simulink model "torque_controller"  (R2014b)
settings: Solver=FixedStepDiscrete  StartTime=0.0  StopTime=inf  FixedStep=sample_time  RelTol=1e-3
StartFcn:
  | tg.sampletime = correctedSampleTime;
libraries: slrtlib x1
settings Model: SimulationMode=external  BufferReuse=off  Creator=wmartin  LastModifiedBy=drl
settings SolverCC: EnableConcurrentExecution=on
settings DataIOCC: LimitDataPoints=off  MaxDataPoints=1e7  SaveFormat=StructureWithTime  SignalLogging=off  DSMLogging=off
settings OptimizationCC: BlockReduction=off  OptimizeBlockIOStorage=off  BufferReuse=off  GlobalBufferReuse=off  ExpressionFolding=off  ExpressionDepthLimit=2147483647  LocalBlockOutputs=off  SimCompilerOptimization=On
settings DebuggingCC: UnderspecifiedInitializationDetection=Classic  MergeDetectMultiDrivingBlocksExec=none  StateNameClashWarn=warning
settings HardwareCC: ProdIntDivRoundTo=Zero  ProdEndianess=LittleEndian  ProdLongLongMode=on  ProdHWDeviceType=Generic->32-bit x86 compatible
settings ModelReferenceCC: UpdateModelReferenceTargets=IfOutOfDate  ModelReferenceNumInstancesAllowed=Single  ModelReferenceMinAlgLoopOccurrences=on
settings RTWCC: SystemTargetFile=slrt.tlc  TemplateMakefile=slrt_default_tmf  Description=Simulink Real-Time  RTWVerbose=off  ProcessScript=slrt_make_rtw_hook  RTWCompilerOptimization=On
settings CodeAppCC: MaxIdLength=256
settings SimulinkRealTimeCC: GeneratePreprocessorConditionals=Disable all  EnableShiftOperators=on  RL32LogBufSizeModifier=1e8

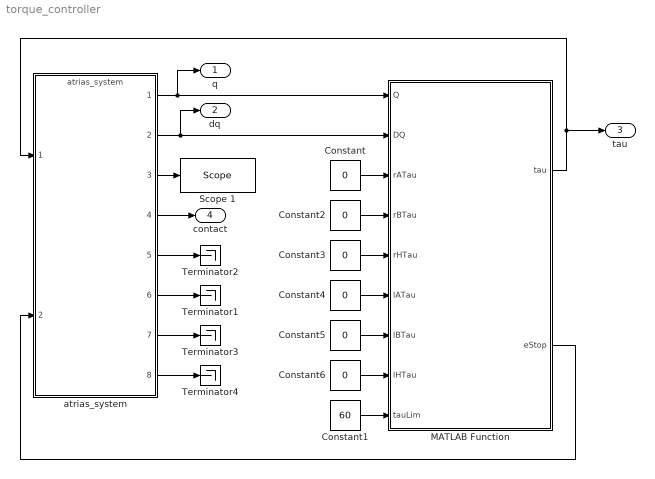
== system torque_controller ==
  Constant{,2..6} (6 alike) : Constant  Value=0
  Constant1 : Constant  Value=60
  MATLAB Function : MATLAB Function  TreatAsAtomicUnit=on
  Scope 1 : slrtlib/Displays and Logging/Scope   scopeno=1  scopetype=Target  autostart=on  viewmode=Graphical sliding  formatstr='%15.6f'  grid=on  ylimits=[0,0]  nosamples=5000  noprepostsamples=0  interleave=1  triggermode=FreeRun  triggersignal=1  trigsignalfromport=off  triggerlevel=0.0  triggerslope=Either  triggerscope=1  triggersample=0  filename=data.dat  mode=Lazy  writesize=512  autorestart=off  dynamicfilemode=off  maxwritefilesize=512*1024^2
  Terminator{1..4} (4 alike) : Terminator
  atrias_system : ModelReference  ModelNameDialog=atrias_system  SimulationMode=Normal  ModelReferenceVersion=1.2412  CopyOfModelName=atrias_system  DefaultDataLogging=on
  q : Outport
  dq : Outport  Port=2
  tau : Outport  Port=3
  contact : Outport  Port=4
  wires:
  atrias_system/2 -> dq/1, MATLAB Function/2(DQ)
  MATLAB Function/1(tau) -> tau/1, atrias_system/1
  MATLAB Function/2(eStop) -> atrias_system/2
  Constant/1 -> MATLAB Function/3(rATau)
  atrias_system/1 -> q/1, MATLAB Function/1(Q)
  Constant1/1 -> MATLAB Function/9(tauLim)
  Constant3/1 -> MATLAB Function/5(rHTau)
  Constant2/1 -> MATLAB Function/4(rBTau)
  Constant4/1 -> MATLAB Function/6(lATau)
  Constant5/1 -> MATLAB Function/7(lBTau)
  Constant6/1 -> MATLAB Function/8(lHTau)
  atrias_system/4 -> contact/1
  atrias_system/6 -> Terminator1/1
  atrias_system/7 -> Terminator3/1
  atrias_system/5 -> Terminator2/1
  atrias_system/8 -> Terminator4/1
  atrias_system/3 -> Scope 1/1

== matlab function torque_controller/MATLAB Function ==
  data: Q input; tau output; DQ input; rATau input; rBTau input; rHTau input; lATau input; lBTau input; lHTau input; eStop output; tauLim input
function [tau, eStop] = torqueController(Q, DQ, rATau, rBTau, rHTau, lATau, lBTau, lHTau, tauLim)
%TRACKINGCONTROLLER Trajectory tracking contoller.
%
% Description:
%
% Notes:
% 	- State indexes (rBl rBm rAl rAm lBl lBm lAl lAm rHm lHm bR bY bP) 
%   - Input indexes (rB rA rH lB lA lH)
    
    % Output vector
    u = [rBTau rATau rHTau lBTau lATau lHTau];
    
    % Set default emergency stop to false
    eStop = false;
    
    % Limit torques to be cautious
	tau = clamp(u, -tauLim, tauLim);

end % sampleController

function b = clamp(a, lim1, lim2)
%CLAMP Clamp value between two values.
	
	% Find which limit is min and max
	aMin = min(lim1);
	aMax = max(lim2);

	% Clamp value between limits
	b = max(min(a, aMax), aMin);
end % clamp
